simulink model "PD_CONTROL"  (R2019b)
settings: Solver=VariableStepAuto  StartTime=0.0  StopTime=t_final  FixedStep=time_step  RelTol=1e-3
undefined symbols (not defined in the file or in its folder): D, P, tau
libraries: cstblocks x1
settings Model: SimulationMode=accelerator  Creator=mchehadeh  LastModifiedBy=aaa_b
settings SolverCC: ZeroCrossAlgorithm=Adaptive
settings DataIOCC: LimitDataPoints=on  SaveFormat=Array  ReturnWorkspaceOutputs=off
settings OptimizationCC: BlockReduction=off  BooleanDataType=off  ExpressionDepthLimit=2147483647  LifeSpan=inf
settings DebuggingCC: SaveWithParameterizedLinksMsg=none  UnderspecifiedInitializationDetection=Classic  MergeDetectMultiDrivingBlocksExec=none  SignalResolutionControl=TryResolveAllWithWarning  IgnoredZcDiagnostic=none  MultiTaskDSMMsg=warning  MultiTaskCondExecSysMsg=none  FcnCallInpInsideContextMsg=warning  StateNameClashWarn=warning  SFUnexpectedBacktrackingDiag=warning  SFNoUnconditionalDefaultTransitionDiag=warning  SFExecutionAtInitializationDiag=none  ArithmeticOperatorsInVariantConditions=warning
settings HardwareCC: ProdBitPerPointer=32  ProdBitPerSizeT=32  ProdBitPerPtrDiffT=32  ProdLargestAtomicFloat=None  ProdIntDivRoundTo=Undefined  ProdEndianess=Unspecified  ProdWordSize=32  ProdHWDeviceType=32-bit Generic  TargetUnknown=on
settings ModelReferenceCC: PropagateSignalLabelsOutOfModel=off
settings SFSimCC: SimUseLocalCustomCode=off  CustomCodeUndefinedFunction=UseInterfaceOnly
settings RTWCC: RTWUseLocalCustomCode=off
settings CodeAppCC: StateflowObjectComments=on
settings GRTTargetCC: TargetLangStandard=C89/C90 (ANSI)  GeneratePreprocessorConditionals=Disable all
settings ConfigComp: CovMetricSettings=dw  CovHtmlReporting=on  CovSaveCumulativeToWorkspaceVar=on  CovSaveSingleToWorkspaceVar=on  CovExternalEMLEnable=off

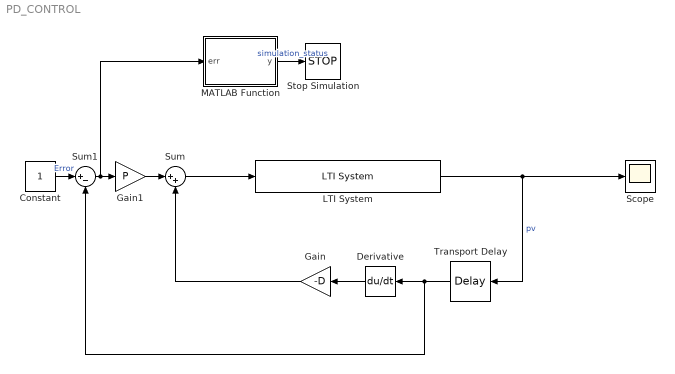
== system PD_CONTROL ==
  Constant : Constant
  Derivative : Derivative
  Gain : Gain  Gain=-D
  Gain1 : Gain  Gain=P
  LTI System : cstblocks/LTI System  sys=g_open  IC=[]
  MATLAB Function : MATLAB Function  TreatAsAtomicUnit=on
  Scope : Scope
  Stop Simulation : Stop
  Sum : Sum  Inputs=|++
  Sum1 : Sum  Inputs=|+-
  Transport Delay : TransportDelay  DelayTime=tau
  wires:
  LTI System/1 -> Transport Delay/1, Scope/1  "pv"
  Transport Delay/1 -> Sum1/2, Derivative/1
  Derivative/1 -> Gain/1
  Gain/1 -> Sum/2
  Sum/1 -> LTI System/1
  Constant/1 -> Sum1/1  "Error"
  Sum1/1 -> MATLAB Function/1(err), Gain1/1
  Gain1/1 -> Sum/1
  MATLAB Function/1(y) -> Stop Simulation/1  "simulation_status"

== matlab function PD_CONTROL/MATLAB Function ==
  data: err input; y output
function y = fcn(err)
if (abs(err)>1000)
    y=1;
else
    y=0;
end
